simulink model "Ordre2"  (R2018a)
settings: Solver=VariableStepAuto  StartTime=0.0  StopTime=10  FixedStep=0.0001  MaxStep=0.001  RelTol=1e-3
libraries: simulink x1
settings Model: Creator=Xavier  LastModifiedBy=Xavier

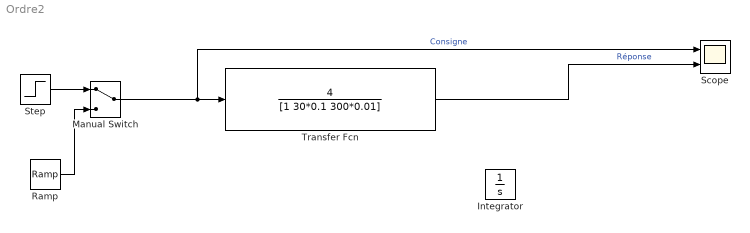
== system Ordre2 ==
  Integrator : Integrator
  Manual Switch : ManualSwitch
  Ramp : simulink/Sources/Ramp  slope=1  start=0  InitialOutput=0
  Scope : Scope  NumInputPorts=2
  Step : Step  SampleTime=0
  Transfer Fcn : TransferFcn  Numerator=[4]  Denominator=[1 30*0.1 300*0.01]
  wires:
  Manual Switch/1 -> Scope/1, Transfer Fcn/1  "Consigne"
  Step/1 -> Manual Switch/1
  Ramp/1 -> Manual Switch/2
  Transfer Fcn/1 -> Scope/2  "Réponse"
